simulink model "testFIB"  (R2019b)
settings: Solver=FixedStepAuto  StartTime=0.0  StopTime=20  RelTol=1e-3
undefined symbols (not defined in the file or in its folder): at, Stuck
libraries: FIBlockLib x2
settings Model: Creator=flata  LastModifiedBy=flata

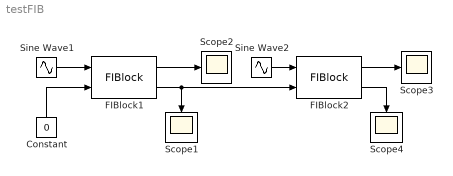
== system testFIB ==
  Constant : Constant  Value=0
  FIBlock1 : FIBlockLib/FIBlock  FIBlockName=1  FInjEnable=on  FaultType=Bias/Offset  FaultValue=2  FaultEvent=Failure probability  EventValue=0.001  FaultEffect=Constant time  EffectValue=1
      settings: SourceProductName=Fault Injection block
  FIBlock2 : FIBlockLib/FIBlock  FIBlockName=2  FInjEnable=on  FaultType=Stuck-at  FaultValue=-3  FaultEvent=Failure probability  EventValue=0  FaultEffect=Constant time  EffectValue=1
      settings: SourceProductName=Fault Injection block
  Scope{1..4} (4 alike) : Scope
  Sine Wave1 : Sin  SampleTime=0
  Sine Wave2 : Sin  SampleTime=0
  wires:
  FIBlock2/1 -> Scope3/1
  FIBlock2/2 -> Scope4/1
  Sine Wave2/1 -> FIBlock2/1
  FIBlock1/1 -> Scope2/1
  Constant/1 -> FIBlock1/2
  Sine Wave1/1 -> FIBlock1/1
  FIBlock1/2 -> FIBlock2/2, Scope1/1
